simulink model "Reference_Generation_Designer"  (R2022a)
settings: Solver=VariableStepAuto  StartTime=0.0  StopTime=100  MaxStep=0.001  RelTol=1e-3
undefined symbols (not defined in the file): Ku, Kv, l, MAX_RADIUS, max_yaw_field, TIRE_ANGLE_MAX, V_target, vehicle_curvature, VELOCITY_MAX_XY
libraries: simulink x1
settings Model: FPTShortcutValueString='{{},{''BaselineRun_4'',1,1,1,''BaselineRun_4'','''',{},''M'',''D'',''''}}'  Creator=Inver  LastModifiedBy=Inver
settings DebuggingCC: SignalRangeChecking=warning

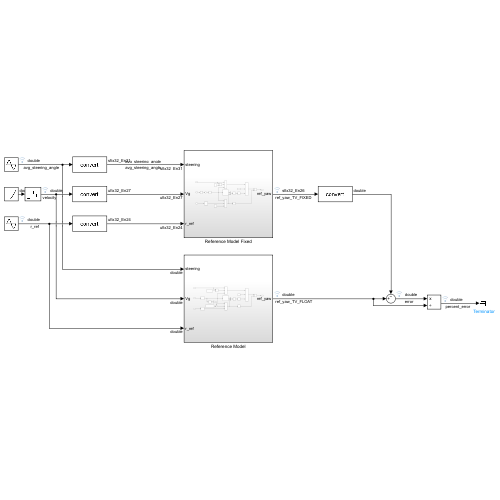
[thumbnail: Simulink's stored preview of the top-level diagram]
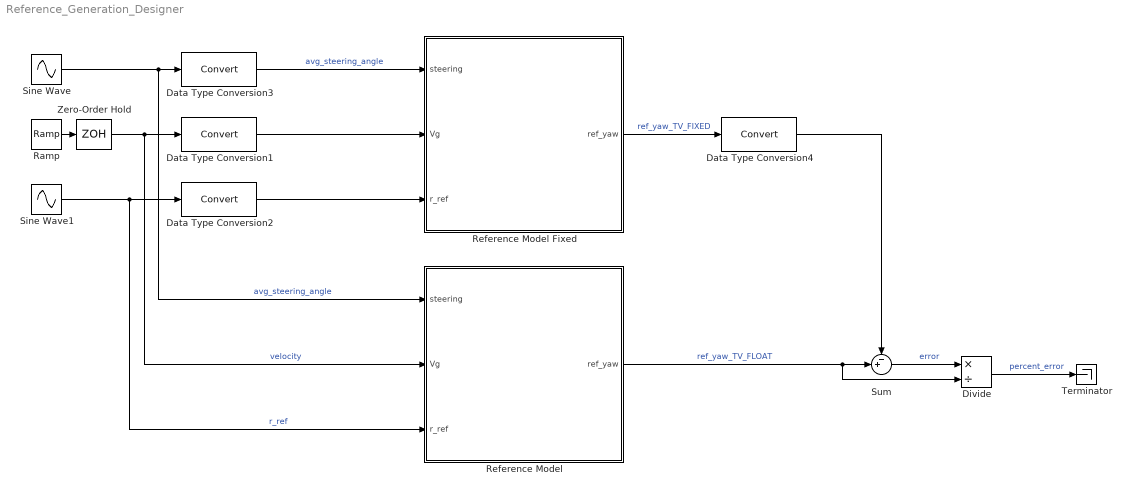
== system Reference_Generation_Designer ==
  Data Type Conversion{1..4} (4 alike) : DataTypeConversion  SaturateOnIntegerOverflow=off  RndMeth=Floor
  Divide : Product  Inputs=*/
  Ramp : simulink/Sources/Ramp  slope=[0 0 VELOCITY_MAX_XY/100]  start=0  InitialOutput=0
  Reference Model : Subsystem
  Reference Model Fixed : Subsystem
  Sine Wave : Sin  Amplitude=[TIRE_ANGLE_MAX 0 0]  Frequency=2*pi  SampleTime=0
  Sine Wave1 : Sin  Amplitude=96  Bias=104  Frequency=2*pi  SampleTime=0
  Sum : Sum  Inputs=-+|
  Terminator : Terminator
  Zero-Order Hold : ZeroOrderHold
  wires:
  Reference Model Fixed/1(ref_yaw) -> Data Type Conversion4/1  "ref_yaw_TV_FIXED"
  Sine Wave1/1 -> Reference Model/3(r_ref), Data Type Conversion2/1  "r_ref"
  Zero-Order Hold/1 -> Reference Model/2(Vg), Data Type Conversion1/1  "velocity"
  Sine Wave/1 -> Reference Model/1(steering), Data Type Conversion3/1  "avg_steering_angle"
  Data Type Conversion1/1 -> Reference Model Fixed/2(Vg)
  Reference Model/1(ref_yaw) -> Divide/2, Sum/2  "ref_yaw_TV_FLOAT"
  Data Type Conversion3/1 -> Reference Model Fixed/1(steering)  "avg_steering_angle"
  Data Type Conversion2/1 -> Reference Model Fixed/3(r_ref)
  Data Type Conversion4/1 -> Sum/1
  Sum/1 -> Divide/1  "error"
  Divide/1 -> Terminator/1  "percent_error"
  Ramp/1 -> Zero-Order Hold/1

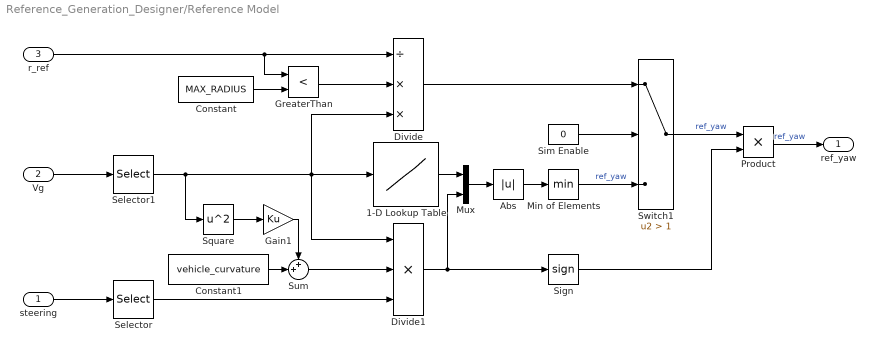
== system Reference_Generation_Designer/Reference Model ==
  steering : Inport  OutDataTypeStr=double  LockScale=on
  Vg : Inport  Port=2  OutDataTypeStr=double  LockScale=on
  r_ref : Inport  Port=3  OutDataTypeStr=double  LockScale=on
  1-D Lookup Table : Lookup_n-D  NumberOfTableDimensions=1  BreakpointsSpecification=Even spacing  BreakpointsForDimension1=V_target  BreakpointsForDimension1FirstPoint=min(V_target)  BreakpointsForDimension1Spacing=V_target(2) - V_target(1)  BreakpointsForDimension1DataTypeStr=double  IndexSearchMethod=Evenly spaced points  BeginIndexSearchUsingPreviousIndexResult=on  Table=max_yaw_field.*Kv  TableDataTypeStr=double  ExtrapMethod=Clip  OutDataTypeStr=double  RndMeth=Simplest
  Abs : Abs  OutDataTypeStr=double  SaturateOnIntegerOverflow=off
  Constant : Constant  Value=MAX_RADIUS  OutDataTypeStr=double
  Constant1 : Constant  Value=vehicle_curvature  OutDataTypeStr=double
  Divide : Product  Inputs=/**  OutDataTypeStr=double
  Divide1 : Product  Inputs=***  OutDataTypeStr=double
  Gain1 : Gain  Gain=Ku
  GreaterThan : RelationalOperator  Operator=<  OutDataTypeStr=boolean  RndMeth=Simplest  InputSameDT=off
  Min of Elements : MinMax  OutDataTypeStr=Inherit: Inherit via back propagation
  Mux : Mux  Inputs=2
  Product : Product  OutDataTypeStr=Inherit: Inherit via back propagation
  Selector : Selector  InputPortWidth=3  IndexOptions=Index vector (dialog)  Indices=1  OutputSizes=1
  Selector1 : Selector  InputPortWidth=3  IndexOptions=Index vector (dialog)  Indices=3  OutputSizes=1
  Sign : Signum
  Sim Enable : Constant  Value=0  OutDataTypeStr=double
  Square : Math  Operator=square
  Sum : Sum  Inputs=++|
  Switch1 : Switch  Criteria=u2 > Threshold  Threshold=1  OutDataTypeStr=Inherit: Inherit via back propagation  SaturateOnIntegerOverflow=off  InputSameDT=off
  ref_yaw : Outport  OutDataTypeStr=double  LockScale=on
  wires:
  Switch1/1 -> Product/1  "ref_yaw"
  Min of Elements/1 -> Switch1/3  "ref_yaw"
  Abs/1 -> Min of Elements/1
  Sim Enable/1 -> Switch1/2
  Mux/1 -> Abs/1
  steering/1 -> Selector/1
  1-D Lookup Table/1 -> Mux/1
  Divide1/1 -> Mux/2, Sign/1
  Product/1 -> ref_yaw/1  "ref_yaw"
  Sign/1 -> Product/2
  Divide/1 -> Switch1/1
  GreaterThan/1 -> Divide/2
  Constant/1 -> GreaterThan/2
  r_ref/1 -> Divide/1, GreaterThan/1
  Selector/1 -> Divide1/3
  Selector1/1 -> Square/1, 1-D Lookup Table/1, Divide/3, Divide1/1
  Vg/1 -> Selector1/1
  Sum/1 -> Divide1/2
  Constant1/1 -> Sum/2
  Square/1 -> Gain1/1
  Gain1/1 -> Sum/1

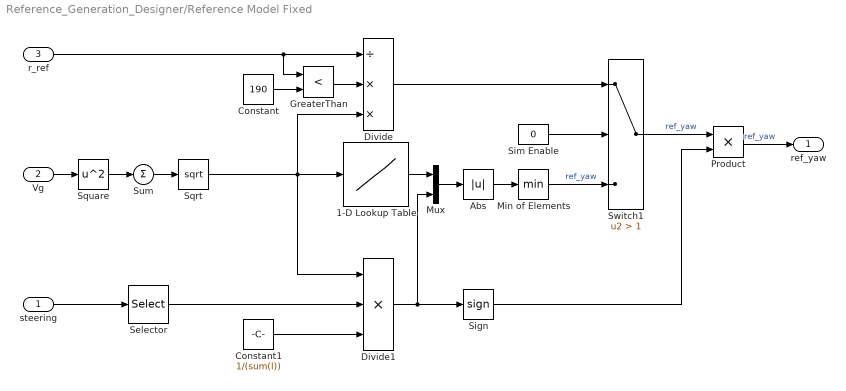
== system Reference_Generation_Designer/Reference Model Fixed ==
  steering : Inport  OutDataTypeStr=fixdt(1,32,31)  LockScale=on
  Vg : Inport  Port=2  OutDataTypeStr=fixdt(0,32,27)  LockScale=on
  r_ref : Inport  Port=3  OutDataTypeStr=fixdt(0,32,24)  LockScale=on
  1-D Lookup Table : Lookup_n-D  NumberOfTableDimensions=1  BreakpointsSpecification=Even spacing  BreakpointsForDimension1=V_target  BreakpointsForDimension1FirstPoint=min(V_target)  BreakpointsForDimension1Spacing=V_target(2) - V_target(1)  BreakpointsForDimension1DataTypeStr=double  IndexSearchMethod=Evenly spaced points  Table=1.5*max_yaw_field  TableDataTypeStr=double  ExtrapMethod=Clip  OutDataTypeStr=fixdt(1,32,26)  RndMeth=Simplest
  Abs : Abs  OutDataTypeStr=Inherit: Inherit via back propagation  SaturateOnIntegerOverflow=off
  Constant : Constant  Value=190  OutDataTypeStr=fixdt(0,16,8)
  Constant1 : Constant  Value=1/(sum(l))  OutDataTypeStr=fixdt(0,16,16)
  Divide : Product  Inputs=/**  OutDataTypeStr=fixdt(1,32,26)
  Divide1 : Product  Inputs=***  OutDataTypeStr=fixdt(1,32,26)
  GreaterThan : RelationalOperator  Operator=<  OutDataTypeStr=boolean  RndMeth=Simplest  InputSameDT=off
  Min of Elements : MinMax  OutDataTypeStr=Inherit: Inherit via back propagation
  Mux : Mux  Inputs=2
  Product : Product  OutDataTypeStr=Inherit: Inherit via back propagation
  Selector : Selector  InputPortWidth=3  IndexOptions=Index vector (dialog)  Indices=1  OutputSizes=1
  Sign : Signum
  Sim Enable : Constant  Value=0  OutDataTypeStr=fixdt(0,4,3)
  Sqrt : Sqrt  OutDataTypeStr=fixdt(0,16,11)
  Square : Math  Operator=square  OutDataTypeStr=fixdt(0,16,6)
  Sum : Sum  Inputs=+  OutDataTypeStr=fixdt(0,16,6)
  Switch1 : Switch  Criteria=u2 > Threshold  Threshold=1  OutDataTypeStr=Inherit: Inherit via back propagation  SaturateOnIntegerOverflow=off  InputSameDT=off
  ref_yaw : Outport  OutDataTypeStr=fixdt(1,32,26)  LockScale=on
  wires:
  Switch1/1 -> Product/1  "ref_yaw"
  Vg/1 -> Square/1
  Min of Elements/1 -> Switch1/3  "ref_yaw"
  Abs/1 -> Min of Elements/1
  Sim Enable/1 -> Switch1/2
  Mux/1 -> Abs/1
  Square/1 -> Sum/1
  Sum/1 -> Sqrt/1
  steering/1 -> Selector/1
  Sqrt/1 -> Divide1/1, Divide/3, 1-D Lookup Table/1
  1-D Lookup Table/1 -> Mux/1
  Divide1/1 -> Mux/2, Sign/1
  Product/1 -> ref_yaw/1  "ref_yaw"
  Sign/1 -> Product/2
  Divide/1 -> Switch1/1
  GreaterThan/1 -> Divide/2
  Constant/1 -> GreaterThan/2
  r_ref/1 -> Divide/1, GreaterThan/1
  Constant1/1 -> Divide1/3
  Selector/1 -> Divide1/2
